simulink library "MarineRoboticsLibEx"  (R2022b)
settings: Solver=VariableStepAuto  StartTime=0.0  StopTime=10.0  RelTol=1e-3
settings Model: Creator=dnad  LastModifiedBy=dnad

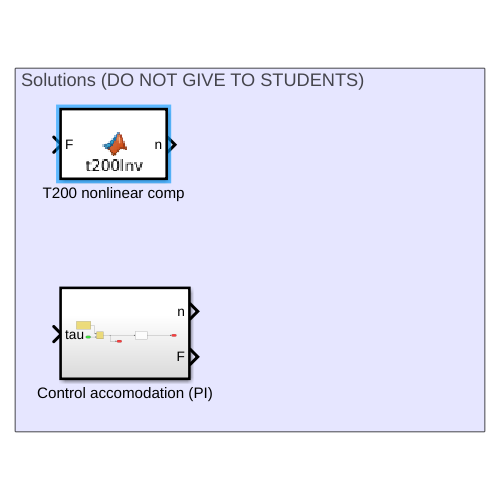
[thumbnail: Simulink's stored preview of the top-level diagram]
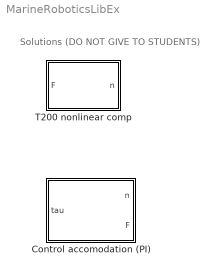
== system MarineRoboticsLibEx ==
  note: Solutions (DO NOT GIVE TO STUDENTS)
  Control accomodation (PI) : Subsystem  TreatAsAtomicUnit=on
  T200 nonlinear comp : MATLAB Function  TreatAsAtomicUnit=on

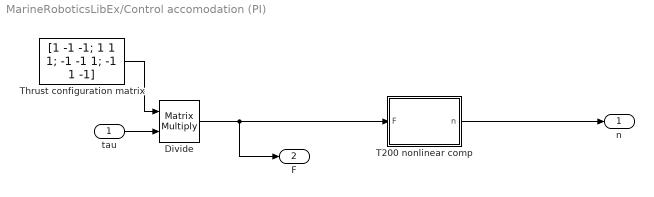
== system MarineRoboticsLibEx/Control accomodation (PI) ==
  tau : Inport
  Divide : Product  Inputs=**  Multiplication=Matrix(*)
  T200 nonlinear comp : MATLAB Function  TreatAsAtomicUnit=on
  Thrust configuration matrix : Constant  Value=|
      | [1 -1 -1;
      | 1 1 1; -1 -1 1; -1 1 -1]
  n : Outport
  F : Outport  Port=2
  wires:
  Divide/1 -> T200 nonlinear comp/1(F), F/1
  Thrust configuration matrix/1 -> Divide/1
  tau/1 -> Divide/2
  T200 nonlinear comp/1(n) -> n/1

== matlab function MarineRoboticsLibEx/Control accomodation (PI)/T200 nonlinear comp ==
  data: F input; n output
function n = t200Inv(F)

% Positive values
ap=0.3252;
bp=0.6596;

% Negative values
an=-0.4509;
bn=-0.7176;

% Clamp into operating range [-1,1] and determine sign for each
n = zeros(size(F));
for i=1:length(F)
    f = F(i);
    fl =min(max(f,-1),1);
    if fl>=0
        n(i) = ap*fl + bp*sqrt(fl);
    elseif fl < 0
        n(i) = -an*fl + bn*sqrt(-fl);
    end
end

== matlab function MarineRoboticsLibEx/T200 nonlinear comp ==
  data: F input; n output
function n = t200Inv(F)

% Positive values
ap=0.3252;
bp=0.6596;

% Negative values
an=-0.4509;
bn=-0.7176;

% Clamp into operating range [-1,1] and determine sign for each
n = zeros(size(F));
for i=1:length(F)
    f = F(i);
    fl =min(max(f,-1),1);
    if fl>=0
        n(i) = ap*fl + bp*sqrt(fl);
    elseif fl < 0
        n(i) = -an*fl + bn*sqrt(-fl);
    end
end
